simulink library "Susp_AxleTA3"  (R2025b)
settings: Solver=VariableStepAuto  StartTime=0.0  StopTime=10.0  RelTol=1e-3
undefined symbols (not defined in the file): Init, Vehicle
libraries: Susp_AxleTA3_Linkage x1, sm_lib x1, Steer_DragLink x1
Description:
  | Component of Simscape Vehicle Templates Library
  | 
  | Copyright 2018-2024 The MathWorks, Inc.
settings Model: Creator=mwalker  LastModifiedBy=smiller
settings SolverCC: AlgebraicLoopSolver=TrustRegion
settings DataIOCC: ReturnWorkspaceOutputs=off
settings DebuggingCC: UnconnectedInputMsg=warning  UnconnectedOutputMsg=warning  UnconnectedLineMsg=warning  ArithmeticOperatorsInVariantConditions=warning
settings ModelReferenceCC: EnableRefExpFcnMdlSchedulingChecks=on
settings SFSimCC: CustomCodeUndefinedFunction=UseInterfaceOnly
settings RTWCC: GPUComputeCapability=3.5

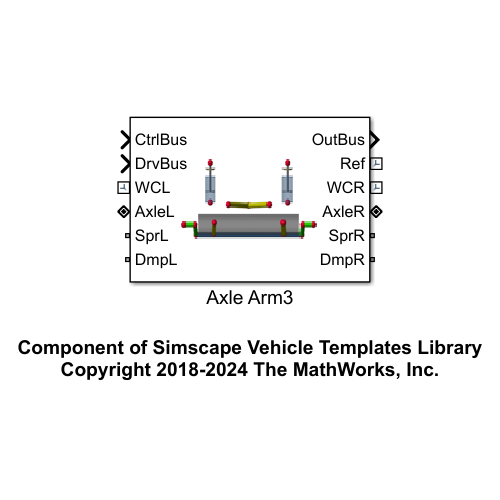
[thumbnail: Simulink's stored preview of the top-level diagram]
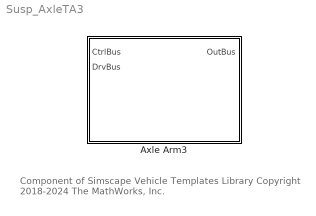
== system Susp_AxleTA3 ==
  note: Component of Simscape Vehicle Templates Library
      | Copyright 2018-2024 The MathWorks, Inc.
  Axle Arm3 : Subsystem  mask(Rigid Axle, Two Trailing Arms, A Arm, with Steering System){Init=Init, Susp=Vehicle.Chassis.SuspA1}
      mask prompts: Init "Initial Values (structure)"; Susp "Susp (structure)"
      mask help: Models a rigid axle connected to the chassis by two trailing arms and an A arm, along with a steering system. The displacement of the springs and dampers are modeled here and the forces are modeled in a separate subsystem.
      mask Display: image('sm_car_vehicle_susp_axleta3_IMAGE.png');

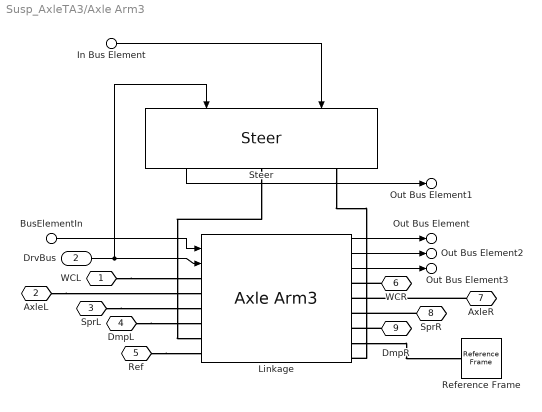
== system Susp_AxleTA3/Axle Arm3 ==
  BusElementIn : Inport  PortName=CtrlBus
  In Bus Element : Inport  PortName=CtrlBus  Element=Steer
  DrvBus : Inport  Port=2
  Linkage : Susp_AxleTA3_Linkage/Axle Arm3  VariantControl=LiveAxle  Init=Init  hp_shock_top=Susp.AxleTA3.Shock.sTop.Value  hp_shock_bot=Susp.AxleTA3.Shock.sBottom.Value  hp_arm_body=Susp.AxleTA3.TrailingArm.sBody.Value  hp_arm_axle=Susp.AxleTA3.TrailingArm.sAxle.Value  hp_arma_body=Susp.AxleTA3.ArmA.sBody.Value  hp_arma_axle=Susp.AxleTA3.ArmA.sAxle.Value  hp_upr_axle=Susp.AxleTA3.Upright.sAxle.Value  hp_steerlink_out=Susp.AxleTA3.SteeringLink.sOutboard.Value  hp_axle_cg=Susp.AxleTA3.Axle.sCG.Value  hp_whl_ctr=Susp.AxleTA3.Upright.sWheelCentre.Value  hp_upr_drag=Susp.AxleTA3.Upright.sDragLink.Value  hp_chassis_bumpstop=Susp.AxleTA3.Bumpstop.sChassis.Value  hp_axle_bumpstop=Susp.AxleTA3.Bumpstop.sAxle.Value  aCaster=Susp.AxleTA3.Upright.aCaster.Value  aKPI=Susp.AxleTA3.Upright.aKPI.Value  axle_mass=Susp.AxleTA3.Axle.m.Value  arm_mass=Susp.AxleTA3.TrailingArm.m.Value  upr_mass=Susp.AxleTA3.Upright.m.Value  steerlink_mass=Susp.AxleTA3.SteeringLink.m.Value  arma_mass=Susp.AxleTA3.ArmA.m.Value  Arm_to_Axle=Susp.AxleTA3.Arm_to_Axle  clr_arm=Visual.UpperArm.clr  opc_arm=Visual.part.opc  radius_arm=Visual.UpperArm.rad  clr_steerlink=Visual.SteeringRack.clr  opc_steerlink=Visual.part.opc  radius_steerlink=Visual.TrackRod.rad  clr_rod=Visual.Pushrod.clr  opc_rod=Visual.part.opc  radius_rod=Visual.Pushrod.rad  clr_conn_links=Visual.hp.clr  opc_conn_links=Visual.hp.opc  size_conn_links=Visual.hp.rad  clr_upr=Visual.Upright.clr  opc_upr=Visual.part.opc  radius_upr=Visual.Upright.rad  piston_mass=Susp.AxleTA3.Shock.mPiston.Value  cyl_mass=Susp.AxleTA3.Shock.mCylinder.Value  shock_xmax=Susp.AxleTA3.Endstop.xMax.Value  shock_xmin=Susp.AxleTA3.Endstop.xMin.Value  Shock_Connection=Susp.AxleTA3.Shock_Connection  Bumpstop_Type=Susp.AxleTA3.Bumpstop.class.Value  bumpstop_height=Susp.AxleTA3.Bumpstop.xHeight.Value  bumpstop_k=Susp.AxleTA3.Bumpstop.K.Value  bumpstop_d=Susp.AxleTA3.Bumpstop.d.Value  bumpstop_xTrans=Susp.AxleTA3.Bumpstop.xTransition.Value  bumpstop_ptcld=Susp.AxleTA3.Bumpstop.sPointCloud.Value
  Reference Frame : sm_lib/Frames and Transforms/Reference Frame
  Steer : Steer_DragLink/Steer  VariantControl=Steer  LabelModeActiveChoice=DragCrossWheelDriven  Steer=Susp.Steer  VariantLabel=Susp.Steer.class.Value
      settings: AttributesFormatString=%<ActiveVariant>
  WCL : PMIOPort  Side=Left
  AxleL : PMIOPort  Port=2  Side=Left
  SprL : PMIOPort  Port=3  Side=Left
  DmpL : PMIOPort  Port=4  Side=Left
  Ref : PMIOPort  Port=5  Side=Right
  WCR : PMIOPort  Port=6  Side=Right
  AxleR : PMIOPort  Port=7  Side=Right
  SprR : PMIOPort  Port=8  Side=Right
  DmpR : PMIOPort  Port=9  Side=Right
  Out Bus Element : Outport  PortName=OutBus  Element=Linkage
  Out Bus Element1 : Outport  PortName=OutBus  Element=Steer
  Out Bus Element2 : Outport  PortName=OutBus  Element=WhlL
  Out Bus Element3 : Outport  PortName=OutBus  Element=WhlR
  wires:
  BusElementIn/1 -> Linkage/1
  Steer/1 -> Out Bus Element1/1
  DrvBus/1 -> Steer/1, Linkage/2
  Linkage/1 -> Out Bus Element/1
  In Bus Element/1 -> Steer/2
  Linkage/2 -> Out Bus Element2/1
  Linkage/3 -> Out Bus Element3/1
  connections:
  AxleL/RConn1 -- Linkage/LConn2
  Steer/RConn1 -- Linkage/LConn5
  DmpL/RConn1 -- Linkage/LConn4
  WCL/RConn1 -- Linkage/LConn1
  SprL/RConn1 -- Linkage/LConn3
  WCR/RConn1 -- Linkage/RConn1
  AxleR/RConn1 -- Linkage/RConn2
  SprR/RConn1 -- Linkage/RConn3
  DmpR/RConn1 -- Linkage/RConn4
  Linkage/RConn5 -- Reference Frame/RConn1
  Steer/RConn2 -- Linkage/RConn6
  Ref/RConn1 -- Linkage/LConn6
